simulink library "mylib"  (R2022b)
settings: Solver=VariableStepAuto  StartTime=0.0  StopTime=10.0  RelTol=1e-3
settings Model: Creator=hessam  LastModifiedBy=hessam

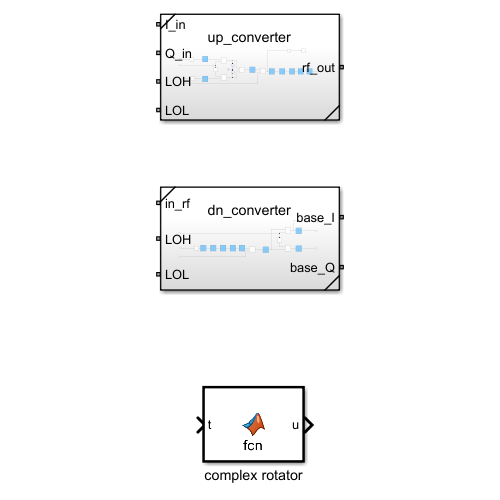
[thumbnail: Simulink's stored preview of the top-level diagram]
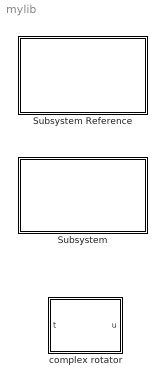
== system mylib ==
  Subsystem : Subsystem  ReferencedSubsystem=dn_converter
      settings: PortSchema="{\"entries\":[{\"content\":{\"sides\":[{\"content\":{\"connectorIds\":[\"LConn3\",\"LConn1\",\"LConn2\"]},\"type\":\"ConnectorPlacement.EquallySpacedRectSide\",\"uuid\":\"8336b51e-e5d8-49cc-804f-7bfb99400ab0\"},{\"content\":{\"connectorIds\":[\"LConn4\",\"LConn5\"],\"side\":\"RIGHT\"},\"type\":\"ConnectorPlacement.EquallySpacedRectSide\",\"uuid\":\"6f005c77-3014-47d2-89f9-41814728faba\"},{\"content\":{\"connectorIds\":[],\"side\":\"TOP\"},\"type\":\"ConnectorPlacement.EquallySpacedRectSide\",\"uuid\":\"edcdef5b-1b73-4458-84fc-72d761e40cdf\"}]},\"type\":\"ConnectorPlacement.EquallySpacedConnector\",\"uuid\":\"3f0b5c66-2f3f-40e5-bb1c-488293219f70\"}],\"packageUris\":[\"http://schema.mathworks.com/mf0/Connector/R2020b\"],\"version\":\"1.0\"}"
  Subsystem Reference : Subsystem  ReferencedSubsystem=up_converter
      settings: PortSchema="{\"entries\":[{\"content\":{\"sides\":[{\"content\":{\"connectorIds\":[\"LConn3\",\"LConn4\",\"LConn2\",\"LConn1\"]},\"type\":\"ConnectorPlacement.EquallySpacedRectSide\",\"uuid\":\"8336b51e-e5d8-49cc-804f-7bfb99400ab0\"},{\"content\":{\"connectorIds\":[\"LConn5\"],\"side\":\"RIGHT\"},\"type\":\"ConnectorPlacement.EquallySpacedRectSide\",\"uuid\":\"6f005c77-3014-47d2-89f9-41814728faba\"},{\"content\":{\"connectorIds\":[],\"side\":\"TOP\"},\"type\":\"ConnectorPlacement.EquallySpacedRectSide\",\"uuid\":\"edcdef5b-1b73-4458-84fc-72d761e40cdf\"}]},\"type\":\"ConnectorPlacement.EquallySpacedConnector\",\"uuid\":\"3f0b5c66-2f3f-40e5-bb1c-488293219f70\"}],\"packageUris\":[\"http://schema.mathworks.com/mf0/Connector/R2020b\"],\"version\":\"1.0\"}"
  complex rotator : MATLAB Function  TreatAsAtomicUnit=on

== matlab function mylib/complex rotator ==
  data: u output; t input
function u   = fcn(t)
   %test of the block
   t=double(t);
   pdb=-12;   %dial input power in dBm 50-ohm reference
   v = sqrt(1/1000*10^(pdb/10));
   f=[1 2 3 4 5 6  ]*455e-5;
   u=v*sum(exp(2.0*3.14*f*t*1j));
